simulink model "zustand_ereignis_umwandlung"  (R2015b)
settings: Solver=FixedStepAuto  StartTime=0.0  StopTime=10.0  RelTol=1e-3
libraries: simulink x1
settings Model: Creator=scco1019  LastModifiedBy=scco1019

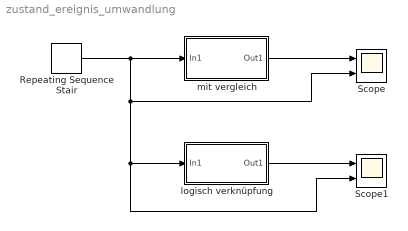
== system zustand_ereignis_umwandlung ==
  Repeating Sequence Stair : simulink/Sources/Repeating Sequence Stair  OutValues=[0 0 1 1 1 1 0 0 1 0 1].'  tsamp=-1  OutMin=[]  OutMax=[]  OutDataTypeStr=double  OutputDataTypeScalingMode=double  OutDataType=fixdt(0,8)  ConRadixGroup=Best Precision: Vector-wise  OutScaling=2^-12
  Scope : Scope  NumInputPorts=2
  Scope1 : Scope  NumInputPorts=2
  logisch verknüpfung : Subsystem
  mit vergleich : Subsystem
  wires:
  Repeating Sequence Stair/1 -> Scope/2, Scope1/2, logisch verknüpfung/1(In1), mit vergleich/1(In1)
  mit vergleich/1(Out1) -> Scope/1
  logisch verknüpfung/1(Out1) -> Scope1/1

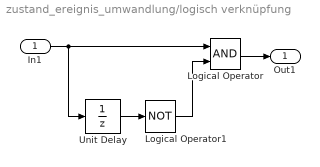
== system zustand_ereignis_umwandlung/logisch verknüpfung ==
  In1 : Inport
  Logical Operator : Logic  AllPortsSameDT=off  OutDataTypeStr=boolean
  Logical Operator1 : Logic  Operator=NOT  AllPortsSameDT=off  OutDataTypeStr=boolean
  Unit Delay : UnitDelay  SampleTime=-1
  Out1 : Outport
  wires:
  In1/1 -> Logical Operator/1, Unit Delay/1
  Logical Operator/1 -> Out1/1
  Unit Delay/1 -> Logical Operator1/1
  Logical Operator1/1 -> Logical Operator/2

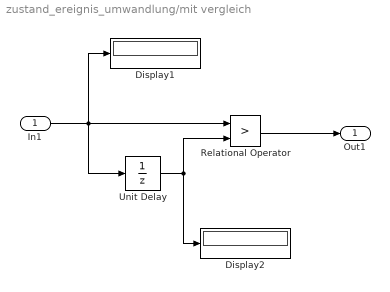
== system zustand_ereignis_umwandlung/mit vergleich ==
  In1 : Inport
  Display1 : Display
  Display2 : Display
  Relational Operator : RelationalOperator  Operator=>  OutDataTypeStr=boolean
  Unit Delay : UnitDelay  SampleTime=-1
  Out1 : Outport
  wires:
  Unit Delay/1 -> Display2/1, Relational Operator/2
  Relational Operator/1 -> Out1/1
  In1/1 -> Display1/1, Unit Delay/1, Relational Operator/1
